simulink model "ex1_b"  (R2020a)
settings: Solver=VariableStepAuto  StartTime=0.0  StopTime=100  RelTol=1e-3
settings Model: Creator=mumun  LastModifiedBy=mumun

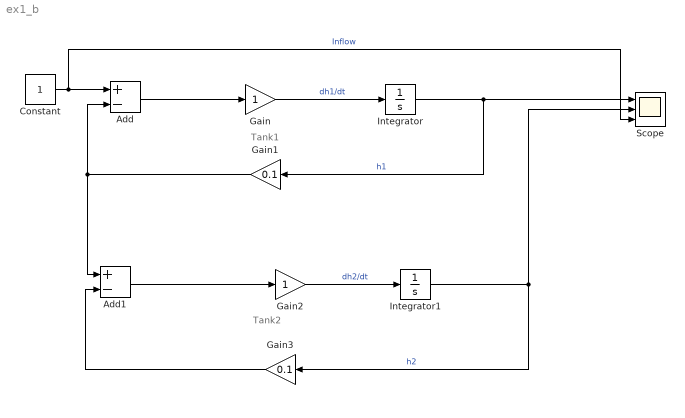
== system ex1_b ==
  note: Tank1
  note: Tank2
  Add : Sum  Inputs=+-
  Add1 : Sum  Inputs=+-
  Constant : Constant
  Gain : Gain
  Gain1 : Gain  Gain=0.1
  Gain2 : Gain
  Gain3 : Gain  Gain=0.1
  Integrator : Integrator  UpperSaturationLimit=2  LowerSaturationLimit=0
  Integrator1 : Integrator  UpperSaturationLimit=2  LowerSaturationLimit=0
  Scope : Scope  NumInputPorts=3
  wires:
  Add/1 -> Gain/1
  Gain/1 -> Integrator/1  "dh1/dt"
  Gain1/1 -> Add1/1, Add/2
  Integrator/1 -> Scope/1, Gain1/1  "h1"
  Add1/1 -> Gain2/1
  Gain2/1 -> Integrator1/1  "dh2/dt"
  Gain3/1 -> Add1/2
  Integrator1/1 -> Gain3/1, Scope/2  "h2"
  Constant/1 -> Scope/3, Add/1  "Inflow"
